simulink model "basic"  (R2016a)
settings: Solver=VariableStepAuto  StartTime=0.0  StopTime=10.0  RelTol=1e-3
values from neighbouring files (symbols this model uses):
  K = lqr(A, B, Qr, Rr)    [LabCEE.m]    (also in fp_ini.m; test.m = [1 2 3 4 5])
  x_0 = [0.1 0 0 0 0]'    [LabCEE.m]    (also in test.m)
undefined symbols (not defined in the file or in its folder): A, B, C, D
settings Model: Creator=ASUS  LastModifiedBy=ASUS

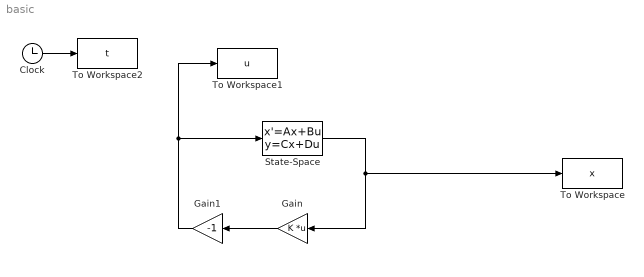
== system basic ==
  Clock : Clock
  Gain : Gain  Gain=K  Multiplication=Matrix(K*u)
  Gain1 : Gain  Gain=-1
  State-Space : StateSpace  A=A  B=B  C=C  D=D  X0=x_0
  To Workspace : ToWorkspace  VariableName=x  SampleTime=-1
  To Workspace1 : ToWorkspace  VariableName=u  SampleTime=-1
  To Workspace2 : ToWorkspace  VariableName=t  SampleTime=-1
  wires:
  State-Space/1 -> Gain/1, To Workspace/1
  Clock/1 -> To Workspace2/1
  Gain/1 -> Gain1/1
  Gain1/1 -> State-Space/1, To Workspace1/1
